simulink model "example_Storage_type2conf"  (R2013b)
settings: Solver=ode45  StartTime=0.0  StopTime=3*3600-2  MaxStep=300  RelTol=1e-3
libraries: carnot x12, simulink x2
settings Model: Creator=drhf  LastModifiedBy=drhf
settings OptimizationCC: ExpressionDepthLimit=2147483647
settings DebuggingCC: StateNameClashWarn=warning
settings GRTTargetCC: CombineOutputUpdateFcns=off  GRTInterface=on

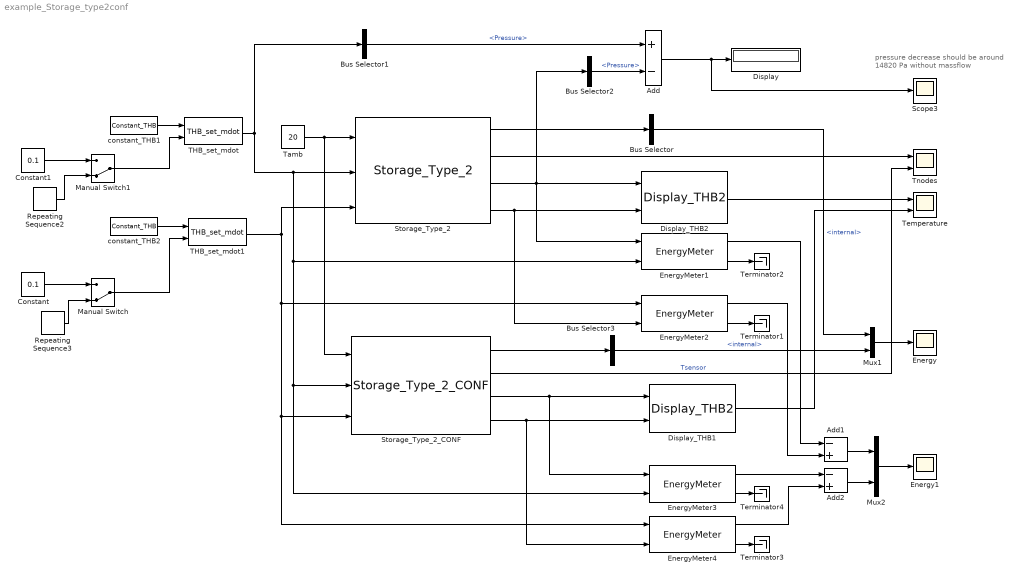
== system example_Storage_type2conf ==
  note: pressure decrease should be
      | around 14820 Pa without massflow
  Add : Sum  Inputs=+-
  Add1 : Sum  Inputs=-+
  Add2 : Sum  Inputs=-+
  Bus Selector : BusSelector  OutputSignals=energy.internal
  Bus Selector1 : BusSelector  OutputSignals=Pressure
  Bus Selector2 : BusSelector  OutputSignals=Pressure
  Bus Selector3 : BusSelector  OutputSignals=energy.internal
  Constant : Constant  Value=0.1
  Constant1 : Constant  Value=0.1
  Display : Display
  Display_THB1 : carnot/Outputs/Display_THB2  t=off  m=on  p=off  id=off  mix=off  d=off
  Display_THB2 : carnot/Outputs/Display_THB2  t=off  m=on  p=off  id=off  mix=off  d=off
  Energy : Scope
  Energy1 : Scope
      settings: SaveName=ScopeData2
  EnergyMeter{1..4} (4 alike) : carnot/Control/EnergyMeter
  Manual Switch : ManualSwitch  CurrentSetting=0
  Manual Switch1 : ManualSwitch  CurrentSetting=0
  Mux1 : Mux  Inputs=2
  Mux2 : Mux  Inputs=2
  Repeating Sequence2 : simulink/Sources/Repeating Sequence  rep_seq_t=[0 1 1.01 2 2.01 2.9 2.91 3.1]*3600  rep_seq_y=[0.12 0.12 0.15 0.15 0.1 0.1 0 0]
  Repeating Sequence3 : simulink/Sources/Repeating Sequence  rep_seq_t=[0 1 1.01 2 2.01 3]*3600  rep_seq_y=[0.12 0.12 0.1 0.1 0.15 0.15]
  Scope3 : Scope
  Storage_Type_2 : carnot/Storage/Thermal/Storage_Type_2  uloss=1  ubot=1  utop=1  cond=1  t0=[10:5:55]  volume=0.3  dia=0.5  pos=standing cylinder  nconnect=2  nodes=10  mpoints=10
  Storage_Type_2_CONF : carnot/Storage/Thermal/Storage_Type_2_CONF  parameterfile=default_Storage  tini=[10:5:55]
  THB_set_mdot : carnot/Source/Simple/THB_set_mdot
  THB_set_mdot1 : carnot/Source/Simple/THB_set_mdot
  Tamb : Constant  Value=20
  Temperature : Scope  NumInputPorts=2
      settings: YMin=-5~-5  YMax=5~5  SaveName=ScopeData4
  Terminator{1..4} (4 alike) : Terminator
  Tnodes : Scope  NumInputPorts=2
      settings: YMin=-5~-5  YMax=5~5  SaveName=ScopeData3
  constant_THB1 : carnot/Source/Simple/Constant_THB  t=55  mdot=0*100/3600  p=1e5  mID=Full Pressure Drop with Static Height  fluid=Water  mix=0  mix2=0  mix3=0  dia=0.02  hgt=0
  constant_THB2 : carnot/Source/Simple/Constant_THB  t=10  mdot=100/3600  p=1e5  mID=Full Pressure Drop with Static Height  fluid=Water  mix=0  mix2=0  mix3=0  dia=0.02  hgt=0
  wires:
  Bus Selector/1 -> Mux1/1  "<internal>"
  Tamb/1 -> Storage_Type_2_CONF/1, Storage_Type_2/1
  THB_set_mdot/1 -> Bus Selector1/1, EnergyMeter3/2, Storage_Type_2_CONF/2, EnergyMeter1/2, Storage_Type_2/2
  THB_set_mdot1/1 -> EnergyMeter4/1, Storage_Type_2_CONF/3, EnergyMeter2/1, Storage_Type_2/3
  Storage_Type_2/1 -> Bus Selector/1
  Storage_Type_2/2 -> Tnodes/1
  Storage_Type_2/3 -> Display_THB2/1, EnergyMeter1/1, Bus Selector2/1
  Storage_Type_2/4 -> Display_THB2/2, EnergyMeter2/2
  Mux1/1 -> Energy/1
  EnergyMeter2/2 -> Terminator1/1
  constant_THB1/1 -> THB_set_mdot/1
  constant_THB2/1 -> THB_set_mdot1/1
  Manual Switch1/1 -> THB_set_mdot/2
  Manual Switch/1 -> THB_set_mdot1/2
  Add/1 -> Display/1, Scope3/1
  Bus Selector1/1 -> Add/1  "<Pressure>"
  Bus Selector2/1 -> Add/2  "<Pressure>"
  Constant/1 -> Manual Switch/1
  Repeating Sequence3/1 -> Manual Switch/2
  Constant1/1 -> Manual Switch1/1
  Repeating Sequence2/1 -> Manual Switch1/2
  EnergyMeter1/2 -> Terminator2/1
  EnergyMeter2/1 -> Add1/2
  EnergyMeter1/1 -> Add1/1
  Storage_Type_2_CONF/2 -> Tnodes/2  "Tsensor"
  Mux2/1 -> Energy1/1
  Storage_Type_2_CONF/3 -> Display_THB1/1, EnergyMeter3/1
  Add1/1 -> Mux2/1
  EnergyMeter3/1 -> Add2/1
  EnergyMeter4/1 -> Add2/2
  Add2/1 -> Mux2/2
  Storage_Type_2_CONF/1 -> Bus Selector3/1
  Bus Selector3/1 -> Mux1/2  "<internal>"
  Storage_Type_2_CONF/4 -> Display_THB1/2, EnergyMeter4/2
  EnergyMeter4/2 -> Terminator3/1
  EnergyMeter3/2 -> Terminator4/1
  Display_THB2/1 -> Temperature/1
  Display_THB1/1 -> Temperature/2
